simulink model "AAITrial"  (R2021a)
settings: Solver=FixedStepAuto  StartTime=0.0  StopTime=10.0  FixedStep=1e-3  RelTol=1e-3  EnableMultiTasking=on
undefined symbols (not defined in the file): D0, D10, D11, D12, D13, D2, D4, D5, D6, D7, D8, D9, PTA0, PTA2, PTB23, PTB9, PTC16, PTC2, PTC3, PTC4, PTD0, PTD1, PTD2, PTD3
libraries: frdmk64flib x15
settings Model: EnablePacing=on  PacingRate=0.250000  ExtModeTrigDuration=5  Creator=Arun Mistry  LastModifiedBy=Arun Mistry
settings OptimizationCC: EnhancedBackFolding=on  PassReuseOutputArgsAs=Individual arguments  ZeroExternalMemoryAtStartup=off  ZeroInternalMemoryAtStartup=off  MaxStackSize=64  OptimizeBlockOrder=speed  DifferentSizesBufferReuse=on  OptimizationCustomize=off  EfficientTunableParamExpr=on
settings DebuggingCC: ParameterTunabilityLossMsg=error
settings HardwareCC: ProdBitPerPointer=32  ProdBitPerSizeT=32  ProdBitPerPtrDiffT=32  ProdLargestAtomicInteger=Long  ProdLargestAtomicFloat=Double  ProdWordSize=32  ProdHWDeviceType=ARM Compatible->ARM Cortex
settings SFSimCC: MATLABDynamicMemAlloc=off
settings RTWCC: SystemTargetFile=ert.tlc  HardwareBoard=NXP FRDM-K64F  TLCOptions="-aInlineSetEventsForThisBaseRateFcn=TLC_FALSE -aSuppressMultiTaskScheduler=TLC_FALSE  -aRateBasedStepFcn=0"  TemplateMakefile=ert_default_tmf  Toolchain=GNU Tools for ARM Embedded Processors
settings CodeAppCC: ForceParamTrailComments=on  IgnoreCustomStorageClasses=off  OperatorAnnotations=on  SimulinkDataObjDesc=on  SFDataObjDesc=on  InsertBlockDesc=on
settings ERTTargetCC: ExtModeTransport=4  ExtModeMexFile=sendToCommService

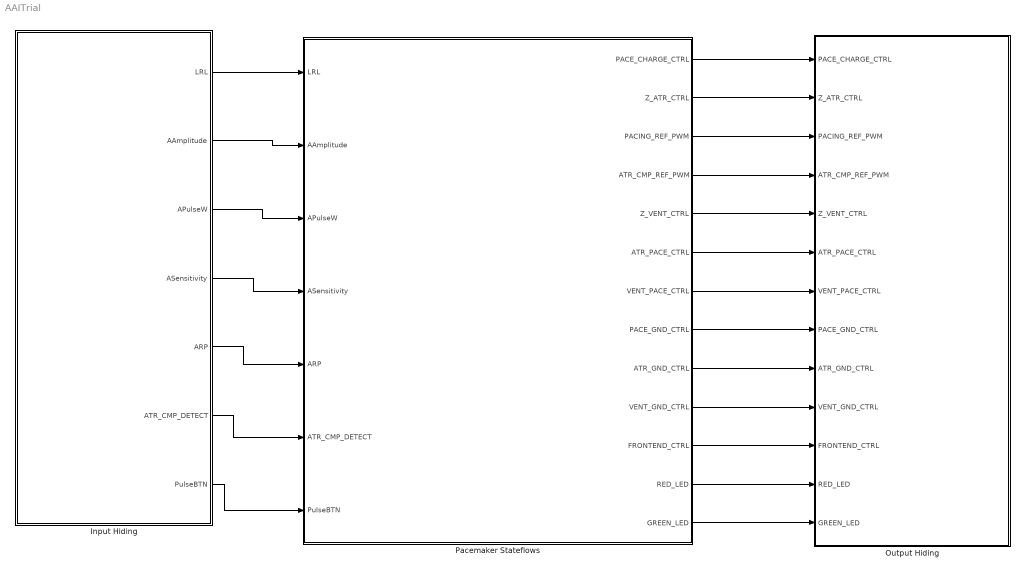
== system AAITrial ==
  Input Hiding : Subsystem
  Output Hiding : Subsystem
  Pacemaker Stateflows : Stateflow chart  TreatAsAtomicUnit=on
  wires:
  Pacemaker Stateflows/4(ATR_CMP_REF_PWM) -> Output Hiding/4(ATR_CMP_REF_PWM)
  Pacemaker Stateflows/2(Z_ATR_CTRL) -> Output Hiding/2(Z_ATR_CTRL)
  Pacemaker Stateflows/10(VENT_GND_CTRL) -> Output Hiding/10(VENT_GND_CTRL)
  Input Hiding/3(APulseW) -> Pacemaker Stateflows/3(APulseW)
  Pacemaker Stateflows/7(VENT_PACE_CTRL) -> Output Hiding/7(VENT_PACE_CTRL)
  Pacemaker Stateflows/12(RED_LED) -> Output Hiding/12(RED_LED)
  Pacemaker Stateflows/13(GREEN_LED) -> Output Hiding/13(GREEN_LED)
  Input Hiding/4(ASensitivity) -> Pacemaker Stateflows/4(ASensitivity)
  Pacemaker Stateflows/11(FRONTEND_CTRL) -> Output Hiding/11(FRONTEND_CTRL)
  Input Hiding/5(ARP) -> Pacemaker Stateflows/5(ARP)
  Input Hiding/1(LRL) -> Pacemaker Stateflows/1(LRL)
  Pacemaker Stateflows/8(PACE_GND_CTRL) -> Output Hiding/8(PACE_GND_CTRL)
  Pacemaker Stateflows/3(PACING_REF_PWM) -> Output Hiding/3(PACING_REF_PWM)
  Pacemaker Stateflows/5(Z_VENT_CTRL) -> Output Hiding/5(Z_VENT_CTRL)
  Input Hiding/2(AAmplitude) -> Pacemaker Stateflows/2(AAmplitude)
  Input Hiding/7(PulseBTN) -> Pacemaker Stateflows/7(PulseBTN)
  Pacemaker Stateflows/9(ATR_GND_CTRL) -> Output Hiding/9(ATR_GND_CTRL)
  Pacemaker Stateflows/6(ATR_PACE_CTRL) -> Output Hiding/6(ATR_PACE_CTRL)
  Input Hiding/6(ATR_CMP_DETECT) -> Pacemaker Stateflows/6(ATR_CMP_DETECT)
  Pacemaker Stateflows/1(PACE_CHARGE_CTRL) -> Output Hiding/1(PACE_CHARGE_CTRL)

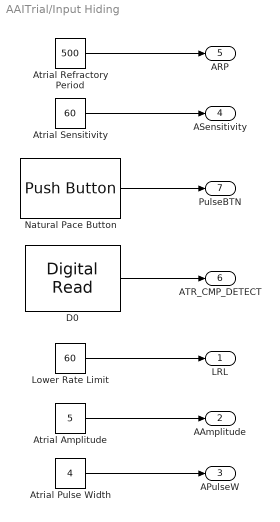
== system AAITrial/Input Hiding ==
  Atrial Amplitude : Constant  Value=5  OutDataTypeStr=double
  Atrial Pulse Width : Constant  Value=4  OutDataTypeStr=double
  Atrial Refractory Period : Constant  Value=500  OutDataTypeStr=double
  Atrial Sensitivity : Constant  Value=60  OutDataTypeStr=double
  D0 : frdmk64flib/Digital Read  Whichpin=PTC16 (D0)  SampleTime=-1
  Lower Rate Limit : Constant  Value=60  OutDataTypeStr=double
  Natural Pace Button : frdmk64flib/Push Button  Whichswitch=SW3  SampleTime1=-1
  LRL : Outport  OutDataTypeStr=double
  AAmplitude : Outport  Port=2  OutDataTypeStr=double
  APulseW : Outport  Port=3  OutDataTypeStr=double
  ASensitivity : Outport  Port=4  OutDataTypeStr=double
  ARP : Outport  Port=5  OutDataTypeStr=double
  ATR_CMP_DETECT : Outport  Port=6  OutDataTypeStr=boolean
  PulseBTN : Outport  Port=7  OutDataTypeStr=boolean
  wires:
  D0/1 -> ATR_CMP_DETECT/1
  Lower Rate Limit/1 -> LRL/1
  Atrial Pulse Width/1 -> APulseW/1
  Atrial Refractory Period/1 -> ARP/1
  Atrial Sensitivity/1 -> ASensitivity/1
  Atrial Amplitude/1 -> AAmplitude/1
  Natural Pace Button/1 -> PulseBTN/1

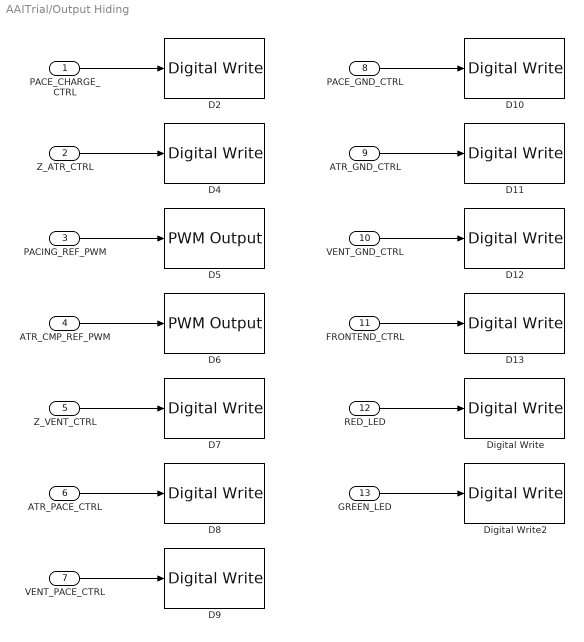
== system AAITrial/Output Hiding ==
  PACE_CHARGE_CTRL : Inport  OutDataTypeStr=double
  Z_ATR_CTRL : Inport  Port=2  OutDataTypeStr=double
  PACING_REF_PWM : Inport  Port=3  OutDataTypeStr=double
  ATR_CMP_REF_PWM : Inport  Port=4  OutDataTypeStr=double
  Z_VENT_CTRL : Inport  Port=5  OutDataTypeStr=double
  ATR_PACE_CTRL : Inport  Port=6  OutDataTypeStr=double
  VENT_PACE_CTRL : Inport  Port=7  OutDataTypeStr=double
  PACE_GND_CTRL : Inport  Port=8  OutDataTypeStr=double
  ATR_GND_CTRL : Inport  Port=9  OutDataTypeStr=double
  VENT_GND_CTRL : Inport  Port=10  OutDataTypeStr=double
  FRONTEND_CTRL : Inport  Port=11  OutDataTypeStr=double
  RED_LED : Inport  Port=12  OutDataTypeStr=double
  GREEN_LED : Inport  Port=13  OutDataTypeStr=double
  D10 : frdmk64flib/Digital Write  Whichpin=PTD0 (D10)
  D11 : frdmk64flib/Digital Write  Whichpin=PTD2 (D11)
  D12 : frdmk64flib/Digital Write  Whichpin=PTD3 (D12)
  D13 : frdmk64flib/Digital Write  Whichpin=PTD1 (D13)
  D2 : frdmk64flib/Digital Write  Whichpin=PTB9 (D2)
  D4 : frdmk64flib/Digital Write  Whichpin=PTB23 (D4)
  D5 : frdmk64flib/PWM Output  Whichpin=PTA2 (D5)  InitialFrequency=2000  InitialDutyCycle=0
  D6 : frdmk64flib/PWM Output  Whichpin=PTC2 (D6)  InitialFrequency=2000  InitialDutyCycle=0
  D7 : frdmk64flib/Digital Write  Whichpin=PTC3 (D7)
  "D8 " : frdmk64flib/Digital Write  Whichpin=PTA0 (D8)
  D9 : frdmk64flib/Digital Write  Whichpin=PTC4 (D9)
  Digital Write : frdmk64flib/Digital Write  Whichpin=RED_LED
  Digital Write2 : frdmk64flib/Digital Write  Whichpin=GREEN_LED
  wires:
  VENT_PACE_CTRL/1 -> D9/1
  ATR_CMP_REF_PWM/1 -> D6/1
  PACE_GND_CTRL/1 -> D10/1
  PACING_REF_PWM/1 -> D5/1
  ATR_GND_CTRL/1 -> D11/1
  ATR_PACE_CTRL/1 -> "D8 "/1
  PACE_CHARGE_CTRL/1 -> D2/1
  FRONTEND_CTRL/1 -> D13/1
  VENT_GND_CTRL/1 -> D12/1
  Z_ATR_CTRL/1 -> D4/1
  Z_VENT_CTRL/1 -> D7/1
  RED_LED/1 -> Digital Write/1
  GREEN_LED/1 -> Digital Write2/1

== stateflow chart AAITrial/Pacemaker Stateflows ==
  state AAI
    entry:
    VENT_PACE_CTRL = 0; VENT_GND_CTRL = 0; PACE_GND_CTRL = 1;
    Z_VENT_CTRL = 0; Z_ATR_CTRL = 0; FRONTEND_CTRL = 1;
    PACING_REF_PWM = AAmplitude*20; ATR_CMP_REF_PWM=ASensitivity;
    state PACE_ATR
      entry:
      PACE_CHARGE_CTRL = 0;
      ATR_GND_CTRL = 0;
      ATR_PACE_CTRL = 1;
      RED_LED = 1;
    state C22_CHARGE
      entry:
      ATR_PACE_CTRL = 0;
      ATR_GND_CTRL = 1;
      PACE_CHARGE_CTRL = 1;
      RED_LED = 0;
    state REFRACTORY
      entry:
      GREEN_LED = 1;
      exit:
      GREEN_LED = 0;
    (default) -> C22_CHARGE
    PACE_ATR -> C22_CHARGE [order 1] : [after(APulseW,msec)]
    C22_CHARGE -> PACE_ATR [order 1] : after((60000/LRL)-APulseW,msec)
    REFRACTORY -> PACE_ATR [order 2] : after(60000/LRL - ARP,msec)
    PACE_ATR -> (junction 151) [order 2] : [ATR_CMP_DETECT == true || PulseBTN == true]
    C22_CHARGE -> (junction 151) [order 2] : [ATR_CMP_DETECT == true || PulseBTN == true]
    (junction 151) -> REFRACTORY : after(ARP,msec){ATR_PACE_CTRL = 0;
        | ATR_GND_CTRL = 1; PACE_CHARGE_CTRL = 1;}
    REFRACTORY -> (junction 151) [order 1] : [ATR_CMP_DETECT == true || PulseBTN == true]
  data: LRL input double; AAmplitude input double; APulseW input double; ASensitivity input double; ARP input double; PACE_CHARGE_CTRL output double; Z_ATR_CTRL output double; PACING_REF_PWM output double; ATR_CMP_REF_PWM output double; Z_VENT_CTRL output double; ATR_PACE_CTRL output double; VENT_PACE_CTRL output double; PACE_GND_CTRL output double; ATR_GND_CTRL output double; VENT_GND_CTRL output double; FRONTEND_CTRL output double; RED_LED output double; GREEN_LED output double; ATR_CMP_DETECT input boolean; PulseBTN input boolean
